simulink model "phan_tich_he_thong_ode"  (R2025a)
settings: Solver=VariableStepAuto  StartTime=0.0  StopTime=80  FixedStep=0.0001  RelTol=1e-3
values from neighbouring files (symbols this model uses):
  B = 0.157142857143    [bien.mat]
  b = 0.8    [bien.mat]
  g = 9.81    [bien.mat]
  L = 0.45    [bien.mat]
  m1 = 1.8    [bien.mat]
  m2 = 0.45    [bien.mat]
undefined symbols (not defined in the file or in its folder): impulseAmplitude, impulseDuration
settings Model: SimulationMode=accelerator  Creator=datng  LastModifiedBy=datng

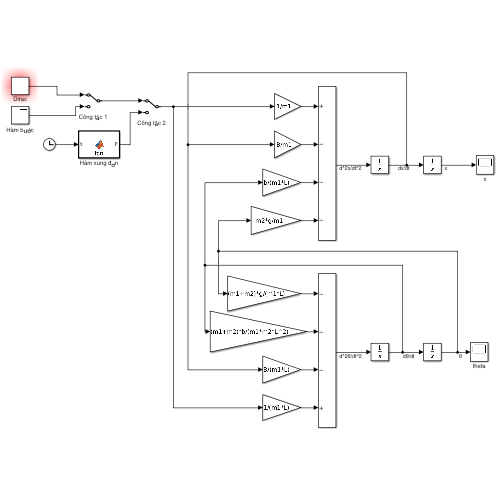
[thumbnail: Simulink's stored preview of the top-level diagram]
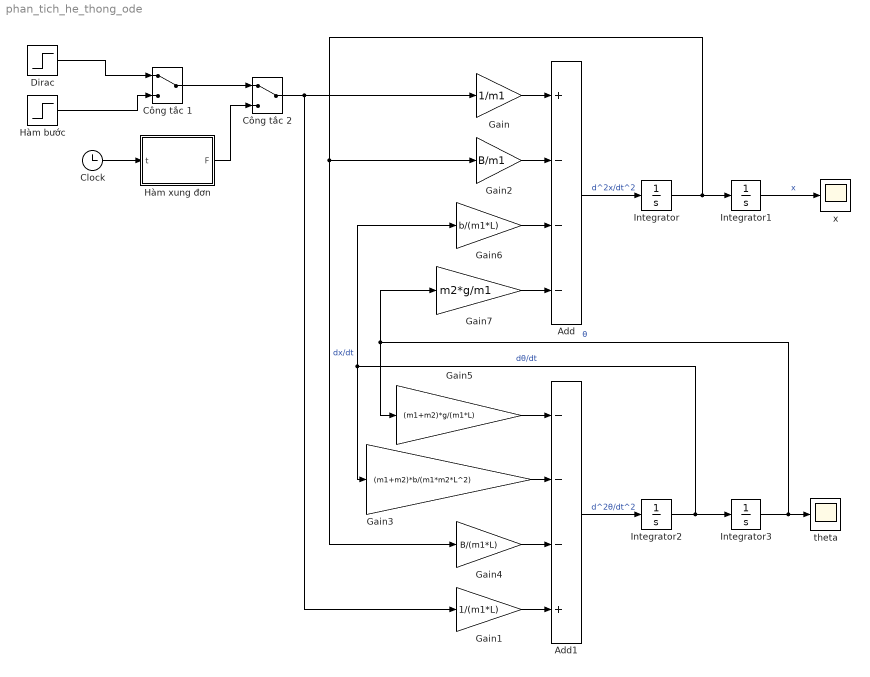
== system phan_tich_he_thong_ode ==
  Add : Sum  Inputs=+---
  Add1 : Sum  Inputs=---+
  Clock : Clock
  Công tắc 1 : ManualSwitch
  Công tắc 2 : ManualSwitch
  Dirac : Step  Time=impulseDuration  Before=impulseAmplitude  After=0  SampleTime=0
  Gain : Gain  Gain=1/m1
  Gain1 : Gain  Gain=1/(m1*L)
  Gain2 : Gain  Gain=B/m1
  Gain3 : Gain  Gain=(m1+m2)*b/(m1*m2*L^2)
  Gain4 : Gain  Gain=B/(m1*L)
  Gain5 : Gain  Gain=(m1+m2)*g/(m1*L)
  Gain6 : Gain  Gain=b/(m1*L)
  Gain7 : Gain  Gain=m2*g/m1
  Hàm bước : Step  Time=0  SampleTime=0
  Hàm xung đơn : MATLAB Function  TreatAsAtomicUnit=on
  Integrator{,1..3} (4 alike) : Integrator
  theta : Scope
      settings: ActiveDisplayYMinimum=-0.18817244724643  ActiveDisplayYMaximum=0.48589962620793009  YLabel=θ (rad)
  x : Scope
      settings: ActiveDisplayYMinimum=-39.765962970374026  ActiveDisplayYMaximum=357.89366673336633  YLabel=x (m)
  wires:
  Gain/1 -> Add/1
  Add/1 -> Integrator/1  "d^2x/dt^2"
  Integrator/1 -> Gain2/1, Gain4/1, Integrator1/1  "dx/dt"
  Gain2/1 -> Add/2
  Gain6/1 -> Add/3
  Gain7/1 -> Add/4
  Gain1/1 -> Add1/4
  Gain5/1 -> Add1/1
  Add1/1 -> Integrator2/1  "d^2θ/dt^2"
  Gain4/1 -> Add1/3
  Gain3/1 -> Add1/2
  Integrator2/1 -> Gain3/1, Gain6/1, Integrator3/1  "dθ/dt"
  Integrator3/1 -> theta/1, Gain5/1, Gain7/1  "θ"
  Hàm bước/1 -> Công tắc 1/2
  Clock/1 -> Hàm xung đơn/1(t)
  Dirac/1 -> Công tắc 1/1
  Hàm xung đơn/1(F) -> Công tắc 2/2
  Công tắc 1/1 -> Công tắc 2/1
  Công tắc 2/1 -> Gain1/1, Gain/1
  Integrator1/1 -> x/1  "x"

== matlab function phan_tich_he_thong_ode/Hàm xung đơn ==
  data: t input; F output
function F = fcn(t)
    if t >= 0 && t <= 5
        F = 10;
    else
        F = 0;
    end
end
